simulink library "nmc"  (R2015b)
settings: Solver=ode45  SolverMode=SingleTasking  StartTime=0.0  StopTime=10.0  RelTol=1e-3
undefined symbols (not defined in the file): c, c_jointstop, CtrlPar_FP_List, CtrlPar_FP_R_List, CtrlPar_LL_List, CtrlPar_St_List, CtrlPar_St_R_List, CtrlPar_Sw_List, CtrlPar_Sw_R_List, CtrlPar_theta0_List, CtrlPar_Tr_List, CtrlPar_Tr_R_List, CtrlPar_VelocityFile_List, D1G_HAT, eref, FmaxBFSH, FmaxGAS, FmaxGLU, FmaxHAB, FmaxHAD, FmaxHAM, FmaxHFL, FmaxRF, FmaxSOL, FmaxTA, FmaxVAS, init_a_tgt, init_a_tgtR, K, leg_l, LongDelay, LongLoopDelay, loptBFSH, loptGAS, loptGLU, loptHAB, loptHAD, loptHAM, loptHFL, loptRF, loptSOL, loptTA, loptVAS, lslackBFSH, lslackGAS, lslackGLU, lslackHAB, lslackHAD, lslackHAM, lslackHFL, lslackRF, lslackSOL, lslackTA, lslackVAS, magnitude, maxLoad_control_List, MidDelay, N, phi12_LowLimit, phi12_UpLimit ... (+96)
libraries: nmc x63, simulink_extras x30, simulink x15, LopesDevelopmentLibrary x3
(part 1 of 10)
settings Model: Creator=efx  LastModifiedBy=brugtjh
settings DataIOCC: SaveFormat=Array
settings OptimizationCC: BlockReduction=off  BooleanDataType=off
settings DebuggingCC: SaveWithParameterizedLinksMsg=none  UnderspecifiedInitializationDetection=Classic  MergeDetectMultiDrivingBlocksExec=none  SignalResolutionControl=TryResolveAllWithWarning  StrictBusMsg=Warning
settings HardwareCC: ProdBitPerPointer=32  ProdLargestAtomicFloat=None  ProdIntDivRoundTo=Undefined  ProdEndianess=Unspecified  ProdWordSize=32  ProdHWDeviceType=32-bit Generic  TargetUnknown=on
settings GRTTargetCC: GeneratePreprocessorConditionals=Disable all
settings ConfigComp: CovModelRefEnable=Off  CovSFcnEnable=off

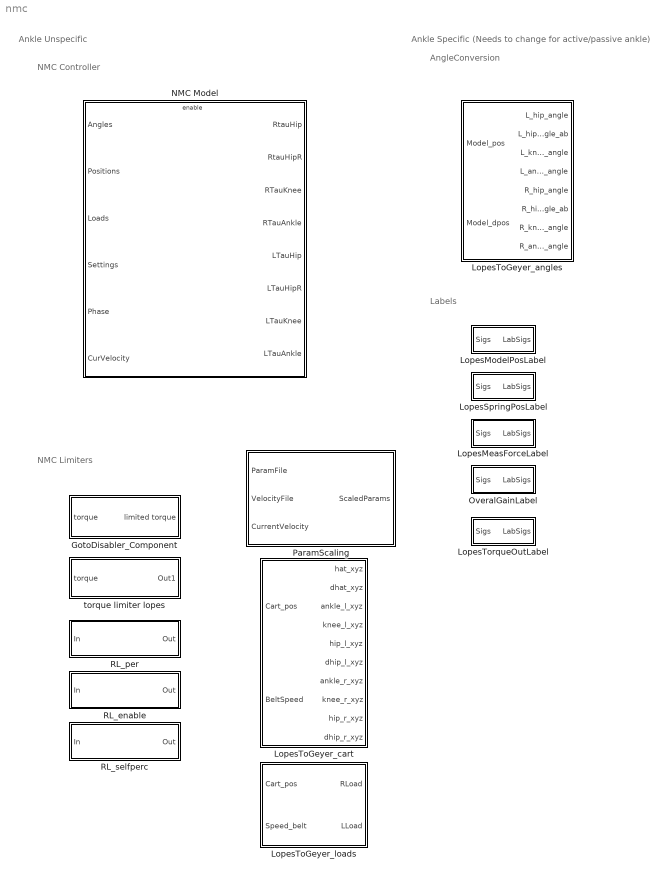
== system nmc ==
  note: Ankle Specific (Needs to change for active/passive ankle)
  note: AngleConversion
  note: NMC Limiters
  note: NMC Controller
  note: Ankle Unspecific
  note: Labels
  GotoDisabler_Component : Subsystem  mask{GotoTag=DisableNMC_Component}
      mask prompts: GotoTag "Simulink:blkprm_prompts:FromGotoTag"
      mask TypeOptions GotoTag: From/GotoTag
  LopesMeasForceLabel : Subsystem
  LopesModelPosLabel : Subsystem
  LopesSpringPosLabel : Subsystem
  LopesToGeyer_angles : Subsystem
  LopesToGeyer_cart : Subsystem
  LopesToGeyer_loads : Subsystem
  LopesTorqueOutLabel : Subsystem
  NMC Model : Subsystem
  OveralGainLabel : Subsystem
  ParamScaling : Subsystem
  RL_enable : Subsystem
  RL_per : Subsystem
  RL_selfperc : Subsystem
  torque limiter lopes : Subsystem  mask{TorqueLimiterPercentage=TorqueLimiterPercentage}
      mask prompts: TorqueLimiterPercentage "Simulink:blkprm_prompts:FromGotoTag"
      mask TypeOptions TorqueLimiterPercentage: From/GotoTag

== system nmc/GotoDisabler_Component ==
  torque : Inport
  Product : Product
  limited torque : Outport
  wires:
  torque/1 -> Product/2
  Product/1 -> limited torque/1
  [DisableNMC_Component] -> Product/1

== system nmc/LopesMeasForceLabel ==
  Sigs : Inport
  AnklePF : Concatenate  NumInputs=1
  Demux : Demux
  HipFlx : Concatenate  NumInputs=1
  KneeFlx : Concatenate  NumInputs=1
  MeasForce - HipAbd : Concatenate  NumInputs=1
  Mux : Mux
  LabSigs : Outport
  wires:
  Demux/3 -> KneeFlx/1
  Demux/2 -> HipFlx/1
  Demux/1 -> MeasForce - HipAbd/1
  HipFlx/1 -> Mux/2  "HipFlx"
  KneeFlx/1 -> Mux/3  "KneeFlx"
  MeasForce - HipAbd/1 -> Mux/1  "MeasForce - HipAbd"
  Sigs/1 -> Demux/1
  Mux/1 -> LabSigs/1
  Demux/4 -> AnklePF/1
  AnklePF/1 -> Mux/4  "AnklePF"

== system nmc/LopesModelPosLabel ==
  Sigs : Inport
  Angle - HipAbd : Concatenate  NumInputs=1
  AnklePF : Concatenate  NumInputs=1
  Demux : Demux
  HipFlx : Concatenate  NumInputs=1
  KneeFlx : Concatenate  NumInputs=1
  Mux : Mux
  LabSigs : Outport
  wires:
  Demux/3 -> KneeFlx/1
  Demux/2 -> HipFlx/1
  Demux/1 -> Angle - HipAbd/1
  HipFlx/1 -> Mux/2  "HipFlx"
  KneeFlx/1 -> Mux/3  "KneeFlx"
  Angle - HipAbd/1 -> Mux/1  "Angle - HipAbd"
  Sigs/1 -> Demux/1
  Mux/1 -> LabSigs/1
  Demux/4 -> AnklePF/1
  AnklePF/1 -> Mux/4  "AnklePF"

== system nmc/LopesSpringPosLabel ==
  Sigs : Inport
  AnklePF : Concatenate  NumInputs=1
  Demux : Demux
  HipFlx : Concatenate  NumInputs=1
  KneeFlx : Concatenate  NumInputs=1
  Mux : Mux
  SpringPos - HipAbd : Concatenate  NumInputs=1
  LabSigs : Outport
  wires:
  Demux/3 -> KneeFlx/1
  Demux/2 -> HipFlx/1
  Demux/1 -> SpringPos - HipAbd/1
  HipFlx/1 -> Mux/2  "HipFlx"
  KneeFlx/1 -> Mux/3  "KneeFlx"
  SpringPos - HipAbd/1 -> Mux/1  "SpringPos - HipAbd"
  Sigs/1 -> Demux/1
  Mux/1 -> LabSigs/1
  Demux/4 -> AnklePF/1
  AnklePF/1 -> Mux/4  "AnklePF"

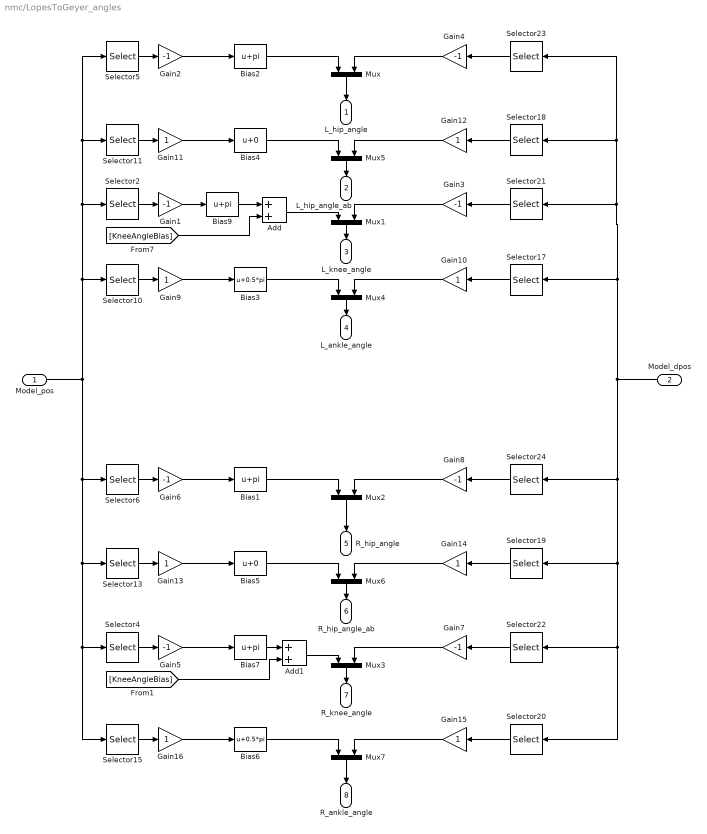
== system nmc/LopesToGeyer_angles ==
  Model_pos : Inport
  Model_dpos : Inport  Port=2
  Add : Sum
  Add1 : Sum
  Bias{1..2,7,9} (4 alike) : Bias  Bias=pi
  Bias3 : Bias  Bias=0.5*pi
  Bias4 : Bias
  Bias5 : Bias
  Bias6 : Bias  Bias=0.5*pi
  Gain{1..8} (8 alike) : Gain  Gain=-1
  Gain{9..16} (8 alike) : Gain
  Mux{,1..7} (8 alike) : Mux  Inputs=2
  Selector10 : Selector  InputPortWidth=SelectorLOPESModelPosSize  IndexOptions=Index vector (dialog)  Indices=[6]  OutputSizes=1
  Selector11 : Selector  InputPortWidth=SelectorLOPESModelPosSize  IndexOptions=Index vector (dialog)  Indices=[3]  OutputSizes=1
  Selector13 : Selector  InputPortWidth=SelectorLOPESModelPosSize  IndexOptions=Index vector (dialog)  Indices=[7]  OutputSizes=1
  Selector15 : Selector  InputPortWidth=SelectorLOPESModelPosSize  IndexOptions=Index vector (dialog)  Indices=[10]  OutputSizes=1
  Selector17 : Selector  InputPortWidth=SelectorLOPESModelPosSize  IndexOptions=Index vector (dialog)  Indices=[6]  OutputSizes=1
  Selector18 : Selector  InputPortWidth=SelectorLOPESModelPosSize  IndexOptions=Index vector (dialog)  Indices=[3]  OutputSizes=1
  Selector19 : Selector  InputPortWidth=SelectorLOPESModelPosSize  IndexOptions=Index vector (dialog)  Indices=[7]  OutputSizes=1
  Selector2 : Selector  InputPortWidth=SelectorLOPESModelPosSize  IndexOptions=Index vector (dialog)  Indices=[5]  OutputSizes=1
  Selector20 : Selector  InputPortWidth=SelectorLOPESModelPosSize  IndexOptions=Index vector (dialog)  Indices=[10]  OutputSizes=1
  Selector21 : Selector  InputPortWidth=SelectorLOPESModelPosSize  IndexOptions=Index vector (dialog)  Indices=[5]  OutputSizes=1
  Selector22 : Selector  InputPortWidth=SelectorLOPESModelPosSize  IndexOptions=Index vector (dialog)  Indices=[9]  OutputSizes=1
  Selector23 : Selector  InputPortWidth=SelectorLOPESModelPosSize  IndexOptions=Index vector (dialog)  Indices=[4]  OutputSizes=1
  Selector24 : Selector  InputPortWidth=SelectorLOPESModelPosSize  IndexOptions=Index vector (dialog)  Indices=[8]  OutputSizes=1
  Selector4 : Selector  InputPortWidth=SelectorLOPESModelPosSize  IndexOptions=Index vector (dialog)  Indices=[9]  OutputSizes=1
  Selector5 : Selector  InputPortWidth=SelectorLOPESModelPosSize  IndexOptions=Index vector (dialog)  Indices=[4]  OutputSizes=1
  Selector6 : Selector  InputPortWidth=SelectorLOPESModelPosSize  IndexOptions=Index vector (dialog)  Indices=[8]  OutputSizes=1
  L_hip_angle : Outport
  L_hip_angle_ab : Outport  Port=2
  L_knee_angle : Outport  Port=3
  L_ankle_angle : Outport  Port=4
  R_hip_angle : Outport  Port=5
  R_hip_angle_ab : Outport  Port=6
  R_knee_angle : Outport  Port=7
  R_ankle_angle : Outport  Port=8
  wires:
  Gain6/1 -> Bias1/1
  Selector6/1 -> Gain6/1
  Gain5/1 -> Bias7/1
  Selector4/1 -> Gain5/1
  Gain2/1 -> Bias2/1
  Selector5/1 -> Gain2/1
  Gain1/1 -> Bias9/1
  Selector2/1 -> Gain1/1
  Bias2/1 -> Mux/1
  Bias1/1 -> Mux2/1
  Selector24/1 -> Gain8/1
  Selector23/1 -> Gain4/1
  Selector21/1 -> Gain3/1
  Gain7/1 -> Mux3/2
  Gain4/1 -> Mux/2
  Gain3/1 -> Mux1/2
  Gain8/1 -> Mux2/2
  Selector22/1 -> Gain7/1
  Mux/1 -> L_hip_angle/1
  Mux1/1 -> L_knee_angle/1
  Mux2/1 -> R_hip_angle/1
  Mux3/1 -> R_knee_angle/1
  Gain9/1 -> Bias3/1
  Selector10/1 -> Gain9/1
  Selector17/1 -> Gain10/1
  Gain10/1 -> Mux4/2
  Gain11/1 -> Bias4/1
  Selector11/1 -> Gain11/1
  Bias4/1 -> Mux5/1
  Selector18/1 -> Gain12/1
  Gain12/1 -> Mux5/2
  Mux5/1 -> L_hip_angle_ab/1
  Gain13/1 -> Bias5/1
  Selector13/1 -> Gain13/1
  Bias5/1 -> Mux6/1
  Selector19/1 -> Gain14/1
  Gain14/1 -> Mux6/2
  Mux6/1 -> R_hip_angle_ab/1
  Model_pos/1 -> Selector2/1, Selector11/1, Selector5/1, Selector10/1, Selector6/1, Selector13/1, Selector15/1, Selector4/1
  Model_dpos/1 -> Selector24/1, Selector19/1, Selector20/1, Selector22/1, Selector17/1, Selector21/1, Selector23/1, Selector18/1
  Gain16/1 -> Bias6/1
  Selector15/1 -> Gain16/1
  Selector20/1 -> Gain15/1
  Gain15/1 -> Mux7/2
  Bias9/1 -> Add/1
  [KneeAngleBias] -> Add/2
  Add/1 -> Mux1/1
  [KneeAngleBias] -> Add1/2
  Bias7/1 -> Add1/1
  Add1/1 -> Mux3/1
  Mux4/1 -> L_ankle_angle/1
  Mux7/1 -> R_ankle_angle/1
  Bias6/1 -> Mux7/1
  Bias3/1 -> Mux4/1

== system nmc/LopesToGeyer_cart ==
  Cart_pos : Inport
  BeltSpeed : Inport  Port=2
  BeltSpeed1 : InportShadow  Port=2
  BeltSpeed2 : InportShadow  Port=2
  Constant : Constant  Value=theta0_control_List
  Constant1 : Constant  Value=CtrlPar_VelocityFile_List
  FilteredDerivative1 : LopesDevelopmentLibrary/Various/FilteredDerivative  w=7*(2*pi)  z=0.7
  FilteredDerivative2 : LopesDevelopmentLibrary/Various/FilteredDerivative  w=7*(2*pi)  z=0.7
  FilteredDerivative3 : LopesDevelopmentLibrary/Various/FilteredDerivative  w=7*(2*pi)  z=0.7
  ParamScaling : nmc/ParamScaling
  Selector1 : Selector  InputPortWidth=21  IndexOptions=Index vector (dialog)  Indices=[1 2 3]  OutputSizes=1
  Selector10 : Selector  InputPortWidth=21  IndexOptions=Index vector (dialog)  Indices=[16 17 18]  OutputSizes=1
  Selector11 : Selector  InputPortWidth=21  IndexOptions=Index vector (dialog)  Indices=[13 14 15]  OutputSizes=1
  Selector2 : Selector  InputPortWidth=7  IndexOptions=Index vector (dialog)  Indices=[2]  OutputSizes=1
  Selector3 : Selector  InputPortWidth=7  IndexOptions=Index vector (dialog)  Indices=[2]  OutputSizes=1
  Selector4 : Selector  InputPortWidth=7  IndexOptions=Index vector (dialog)  Indices=[2]  OutputSizes=1
  Selector5 : Selector  InputPortWidth=21  IndexOptions=Index vector (dialog)  Indices=[10 11 12]  OutputSizes=1
  Selector6 : Selector  InputPortWidth=21  IndexOptions=Index vector (dialog)  Indices=[7 8 9]  OutputSizes=1
  Selector7 : Selector  InputPortWidth=21  IndexOptions=Index vector (dialog)  Indices=[4 5 6]  OutputSizes=1
  Selector9 : Selector  InputPortWidth=21  IndexOptions=Index vector (dialog)  Indices=[19 20 21]  OutputSizes=1
  Subsystem : Subsystem
  Subsystem1 : Subsystem
  Subsystem2 : Subsystem
  Subsystem7 : Subsystem
  hat_xyz : Outport
  dhat_xyz : Outport  Port=2
  ankle_l_xyz : Outport  Port=3
  knee_l_xyz : Outport  Port=4
  hip_l_xyz : Outport  Port=5
  dhip_l_xyz : Outport  Port=6
  ankle_r_xyz : Outport  Port=7
  knee_r_xyz : Outport  Port=8
  hip_r_xyz : Outport  Port=9
  dhip_r_xyz : Outport  Port=10
  wires:
  Cart_pos/1 -> Selector10/1, Selector11/1, Selector9/1, Selector1/1, Selector5/1, Selector6/1, Selector7/1
  FilteredDerivative2/1 -> Subsystem7/1(1)
  FilteredDerivative1/1 -> Subsystem1/1(1)
  Selector6/1 -> knee_l_xyz/1
  Selector7/1 -> hip_l_xyz/1, FilteredDerivative1/1
  Selector5/1 -> ankle_l_xyz/1
  Selector9/1 -> ankle_r_xyz/1
  Selector10/1 -> knee_r_xyz/1
  Selector1/1 -> Subsystem/1(Pelvis_XYZ)
  Selector11/1 -> hip_r_xyz/1, FilteredDerivative3/1
  Subsystem7/1(2) -> dhat_xyz/1
  Subsystem1/1(2) -> dhip_l_xyz/1
  Subsystem2/1(2) -> dhip_r_xyz/1
  BeltSpeed/1 -> Selector4/1
  BeltSpeed1/1 -> Selector2/1
  Selector2/1 -> Subsystem1/2(BeltSpeed)
  BeltSpeed2/1 -> Selector3/1
  Selector3/1 -> Subsystem2/2(BeltSpeed)
  FilteredDerivative3/1 -> Subsystem2/1(1)
  Subsystem/1(HAT_XYZ) -> hat_xyz/1, FilteredDerivative2/1
  Constant/1 -> ParamScaling/1
  Constant1/1 -> ParamScaling/2
  Selector4/1 -> Subsystem7/2(BeltSpeed), ParamScaling/3
  ParamScaling/1 -> Subsystem/2(BodyAngle)

== system nmc/LopesToGeyer_loads ==
  Cart_pos : Inport
  "Speed_belt " : Inport  Port=2
  Add : Sum  Inputs=+-
  Add1 : Sum  Inputs=+-
  Add2 : Sum  Inputs=-+
  Bias : Bias  Bias=0.5*pi
  COPz : Selector  InputPortWidth=7  IndexOptions=Index vector (dialog)  Indices=[6]  OutputSizes=1
  Constant : Constant  Value=maxLoad_control_List
  Constant1 : Constant  Value=CtrlPar_VelocityFile_List
  Divide : Product  Inputs=**
  Divide1 : Product  Inputs=**
  Left_Ankle_z : Selector  InputPortWidth=21  IndexOptions=Index vector (dialog)  Indices=[12]  OutputSizes=1
  MeasuredSpeed : Selector  InputPortWidth=7  IndexOptions=Index vector (dialog)  Indices=[2]  OutputSizes=1
  ParamScaling : nmc/ParamScaling
  Right_Ankle_z : Selector  InputPortWidth=21  IndexOptions=Index vector (dialog)  Indices=[21]  OutputSizes=1
  SafeDivide : Subsystem
      mask Display:
      | port_label('input',1,'/')
      | port_label('input',2,'X')
      | port_label('output',1,'')
  SafeDivide1 : Subsystem
      mask Display:
      | port_label('input',1,'/')
      | port_label('input',2,'X')
      | port_label('output',1,'')
  Saturation : Saturate  UpperLimit=inf  LowerLimit=0
  Saturation1 : Saturate  UpperLimit=inf  LowerLimit=0
  "RLoad " : Outport
  LLoad : Outport  Port=2
  wires:
  Cart_pos/1 -> Left_Ankle_z/1, Right_Ankle_z/1
  "Speed_belt "/1 -> COPz/1, MeasuredSpeed/1
  Left_Ankle_z/1 -> Add1/1, Add/1
  Right_Ankle_z/1 -> Add2/1, Add/2
  COPz/1 -> Add2/2, Add1/2
  Add/1 -> SafeDivide1/1(Denominator), SafeDivide/1(Denominator)
  Add1/1 -> SafeDivide1/2(Numerator)
  SafeDivide1/1(Out) -> Divide/2
  SafeDivide/1(Out) -> Divide1/2
  Divide1/1 -> Saturation1/1
  Divide/1 -> Saturation/1
  Saturation/1 -> "RLoad "/1
  Saturation1/1 -> LLoad/1
  Add2/1 -> SafeDivide/2(Numerator)
  Constant/1 -> ParamScaling/1
  ParamScaling/1 -> Divide1/1, Divide/1
  Constant1/1 -> ParamScaling/2
  MeasuredSpeed/1 -> ParamScaling/3

== system nmc/LopesTorqueOutLabel ==
  Sigs : Inport
  AnklePF : Concatenate  NumInputs=1
  Demux : Demux
  HipFlx : Concatenate  NumInputs=1
  KneeFlx : Concatenate  NumInputs=1
  Mux : Mux
  TorqueOut - HipAbd : Concatenate  NumInputs=1
  LabSigs : Outport
  wires:
  Demux/3 -> KneeFlx/1
  Demux/2 -> HipFlx/1
  Demux/1 -> TorqueOut - HipAbd/1
  HipFlx/1 -> Mux/2  "HipFlx"
  KneeFlx/1 -> Mux/3  "KneeFlx"
  TorqueOut - HipAbd/1 -> Mux/1  "TorqueOut - HipAbd"
  Sigs/1 -> Demux/1
  Mux/1 -> LabSigs/1
  Demux/4 -> AnklePF/1
  AnklePF/1 -> Mux/4  "AnklePF"

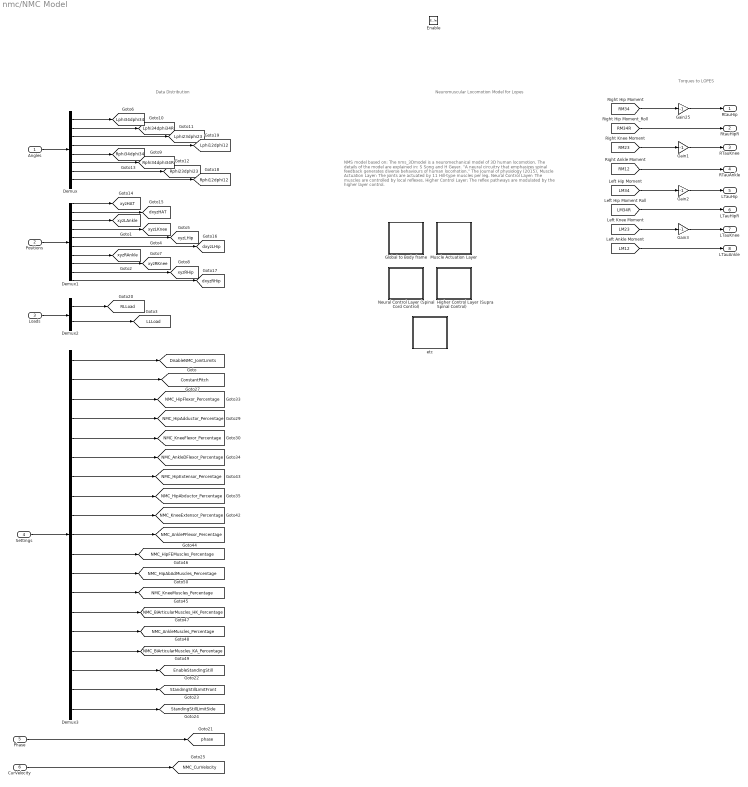
== system nmc/NMC Model ==
  note: Neuromuscular Locomotion Model for Lopes
  note: NMS model based on:
      | The nms_3Dmodel is a neuromechanical model of 3D human locomotion.
      | The details of the model are explained in:
      | S Song and H Geyer. "A neural circuitry that emphasizes spinal feedback
      | generates diverse behaviours of human locomotion." The Journal of physiology (2015).
      |
      | Muscle Actuation Layer:
      | The joints are actuated by 11 Hill-type muscles per leg.
      |
      | Neural Control Layer:
      | The muscles are controlled by local reflexes.
      |
      | Higher Control Layer:
      | The reflex pathways are modulated by the higher layer control.
  note: Data Distribution
  note: Torques to LOPES
  Angles : Inport
  Positions : Inport  Port=2
  Loads : Inport  Port=3
  Settings : Inport  Port=4
  Phase : Inport  Port=5
  CurVelocity : Inport  Port=6
  Enable : EnablePort  StatesWhenEnabling=reset
  Demux : Demux  Outputs=8
  Demux1 : Demux  Outputs=10
  Demux2 : Demux  Outputs=2
  Demux3 : Demux  Outputs=19
  Gain{1..3,25} (4 alike) : Gain  Gain=-1
  Global to Body frame : Subsystem
  Higher Control Layer (Supra Spinal Control) : Subsystem
  Muscle Actuation Layer : Subsystem
  Neural Control Layer (Spinal Cord Control) : Subsystem
  etc : Subsystem
  RtauHip : Outport
  RtauHipR : Outport  Port=2
  RTauKnee : Outport  Port=3
  RTauAnkle : Outport  Port=4
  LTauHip : Outport  Port=5
  LTauHipR : Outport  Port=6
  LTauKnee : Outport  Port=7
  LTauAnkle : Outport  Port=8
  tag scope: ConstantPitch=global, DisableNMC_JointLimits=global, EnableStandingStill=global, LLLoad=global, Lphi12dphi12=global, Lphi23dphi23=global, Lphi34dphi34=global, Lphi34dphi34R=global, NMC_AnkleDFlexor_Percentage=global, NMC_AnkleMuscles_Percentage=global, NMC_AnklePFlexor_Percentage=global, NMC_BiArticularMuscles_HK_Percentage=global, NMC_BiArticularMuscles_KA_Percentage=global, NMC_CurVelocity=global, NMC_HipAbAdMuscles_Percentage=global, NMC_HipAbductor_Percentage=global, NMC_HipAdductor_Percentage=global, NMC_HipExtensor_Percentage=global, NMC_HipFEMuscles_Percentage=global, NMC_HipFlexor_Percentage=global, NMC_KneeExtensor_Percentage=global, NMC_KneeFlexor_Percentage=global, NMC_KneeMuscles_Percentage=global, RLLoad=global, Rphi12dphi12=global, Rphi23dphi23=global, Rphi34dphi34=global, Rphi34dphi34R=global, StandingStillLimitFront=global, StandingStillLimitSide=global, dxyzHAT=global, dxyzLHip=global, dxyzRHip=global, phase=global, xyzHAT=global, xyzLAnkle=global, xyzLHip=global, xyzLKnee=global, xyzRAnkle=global, xyzRHip=global, xyzRKnee=global
  wires:
  [RM34] -> Gain25/1
  [RM23] -> Gain1/1
  [LM34] -> Gain2/1
  [LM23] -> Gain3/1
  Angles/1 -> Demux/1
  Demux/1 -> [Lphi34dphi34]
  Demux/5 -> [Rphi34dphi34]
  Demux/6 -> [Rphi34dphi34R]
  Demux/7 -> [Rphi23dphi23]
  Demux/8 -> [Rphi12dphi12]
  Demux/2 -> [Lphi34dphi34R]
  Demux/3 -> [Lphi23dphi23]
  Demux/4 -> [Lphi12dphi12]
  Positions/1 -> Demux1/1
  Demux1/1 -> [xyzHAT]
  Demux1/2 -> [dxyzHAT]
  Loads/1 -> Demux2/1
  Demux2/1 -> [RLLoad]
  Demux2/2 -> [LLLoad]
  Demux1/3 -> [xyzLAnkle]
  Demux1/4 -> [xyzLKnee]
  Demux1/5 -> [xyzLHip]
  Demux1/6 -> [dxyzLHip]
  Demux1/7 -> [xyzRAnkle]
  Demux1/8 -> [xyzRKnee]
  Demux1/9 -> [xyzRHip]
  Demux1/10 -> [dxyzRHip]
  [RM34R] -> RtauHipR/1
  [RM12] -> RTauAnkle/1
  [LM34R] -> LTauHipR/1
  [LM12] -> LTauAnkle/1
  Phase/1 -> [phase]
  Settings/1 -> Demux3/1
  Demux3/2 -> [ConstantPitch]
  Demux3/1 -> [DisableNMC_JointLimits]
  Demux3/15 -> [NMC_AnkleMuscles_Percentage]
  Demux3/13 -> [NMC_KneeMuscles_Percentage]
  Demux3/14 -> [NMC_BiArticularMuscles_HK_Percentage]
  Demux3/16 -> [NMC_BiArticularMuscles_KA_Percentage]
  Demux3/12 -> [NMC_HipAbAdMuscles_Percentage]
  Demux3/11 -> [NMC_HipFEMuscles_Percentage]
  Demux3/10 -> [NMC_AnklePFlexor_Percentage]
  Demux3/9 -> [NMC_KneeExtensor_Percentage]
  Demux3/8 -> [NMC_HipAbductor_Percentage]
  Demux3/7 -> [NMC_HipExtensor_Percentage]
  Demux3/6 -> [NMC_AnkleDFlexor_Percentage]
  Demux3/5 -> [NMC_KneeFlexor_Percentage]
  Demux3/4 -> [NMC_HipAdductor_Percentage]
  Demux3/3 -> [NMC_HipFlexor_Percentage]
  Gain25/1 -> RtauHip/1
  Gain1/1 -> RTauKnee/1
  Gain2/1 -> LTauHip/1
  Gain3/1 -> LTauKnee/1
  Demux3/17 -> [EnableStandingStill]
  Demux3/18 -> [StandingStillLimitFront]
  Demux3/19 -> [StandingStillLimitSide]
  CurVelocity/1 -> [NMC_CurVelocity]

== system nmc/OveralGainLabel ==
  Sigs : Inport
  AnklePF : Concatenate  NumInputs=1
  Demux : Demux
  HipFlx : Concatenate  NumInputs=1
  KneeFlx : Concatenate  NumInputs=1
  Mux : Mux
  OveralGain - HipAbd : Concatenate  NumInputs=1
  LabSigs : Outport
  wires:
  Demux/3 -> KneeFlx/1
  Demux/2 -> HipFlx/1
  Demux/1 -> OveralGain - HipAbd/1
  HipFlx/1 -> Mux/2  "HipFlx"
  KneeFlx/1 -> Mux/3  "KneeFlx"
  OveralGain - HipAbd/1 -> Mux/1  "OveralGain - HipAbd"
  Sigs/1 -> Demux/1
  Mux/1 -> LabSigs/1
  Demux/4 -> AnklePF/1
  AnklePF/1 -> Mux/4  "AnklePF"

== system nmc/ParamScaling ==
  ParamFile : Inport
  VelocityFile : Inport  Port=2
  CurrentVelocity : Inport  Port=3
  ScalerFull : MATLAB Function
      settings: MinAlgLoopOccurrences=on
  ScaledParams : Outport
  wires:
  ScalerFull/1(ScaledParam) -> ScaledParams/1
  ParamFile/1 -> ScalerFull/1(ParamFile)
  VelocityFile/1 -> ScalerFull/2(VelocityFile)
  CurrentVelocity/1 -> ScalerFull/3(Velocity)

== system nmc/RL_enable ==
  In : Inport
  Gain : Gain  Gain=-1
  Gain1 : Gain  Gain=0.01
  Rate Limiter Dynamic : simulink/Discontinuities/Rate Limiter Dynamic
  Out : Outport
  wires:
  Gain1/1 -> Rate Limiter Dynamic/1, Gain/1
  Gain/1 -> Rate Limiter Dynamic/3
  [RateLimiterPercentage] -> Gain1/1
  In/1 -> Rate Limiter Dynamic/2
  Rate Limiter Dynamic/1 -> Out/1

== system nmc/RL_per ==
  In : Inport
  Gain : Gain  Gain=-1
  Rate Limiter Dynamic : simulink/Discontinuities/Rate Limiter Dynamic
  Out : Outport
  wires:
  Rate Limiter Dynamic/1 -> Out/1
  In/1 -> Rate Limiter Dynamic/2
  [RateLimiterPercentage] -> Gain/1, Rate Limiter Dynamic/1
  Gain/1 -> Rate Limiter Dynamic/3

== system nmc/RL_selfperc ==
  In : Inport
  Constant : Constant  Value=0
  Gain : Gain  Gain=-1
  MinMax Running Resettable : simulink/Math Operations/MinMax Running Resettable  Function=max  vinit=0.0
  PercToPoint : Gain  Gain=0.01
  Product : Product
  Rate Limiter Dynamic : simulink/Discontinuities/Rate Limiter Dynamic
  Out : Outport
  wires:
  Constant/1 -> MinMax Running Resettable/2
  MinMax Running Resettable/1 -> Rate Limiter Dynamic/1, Gain/1
  Gain/1 -> Rate Limiter Dynamic/3
  In/1 -> Product/2, Rate Limiter Dynamic/2
  Rate Limiter Dynamic/1 -> Out/1
  [RateLimiterPercentage] -> PercToPoint/1
  PercToPoint/1 -> Product/1
  Product/1 -> MinMax Running Resettable/1

== system nmc/torque limiter lopes ==
  torque : Inport
  Gain1 : Gain  Gain=0.01
  Product1 : Product
  Out1 : Outport
  wires:
  Product1/1 -> Out1/1
  torque/1 -> Product1/2
  [TorqueLimiterPercentage] -> Gain1/1
  Gain1/1 -> Product1/1

== system nmc/LopesToGeyer_cart/Subsystem ==
  Pelvis_XYZ : Inport
  BodyAngle : Inport  Port=2
  Add : Sum
  Add1 : Sum
  Demux : Demux  Outputs=3
  Gain : Gain  Gain=D1G_HAT
  Gain1 : Gain
  Gain2 : Gain  Gain=D1G_HAT
  Mux : Mux  Inputs=3
  Trigonometric Function : Trigonometry
  Trigonometric Function1 : Trigonometry  Operator=cos
  HAT_XYZ : Outport
  wires:
  Mux/1 -> HAT_XYZ/1
  Add1/1 -> Mux/2
  Demux/3 -> Gain1/1
  Pelvis_XYZ/1 -> Demux/1
  Demux/2 -> Add1/2
  Demux/1 -> Add/2
  Gain1/1 -> Mux/3
  Add/1 -> Mux/1
  BodyAngle/1 -> Trigonometric Function1/1, Trigonometric Function/1
  Trigonometric Function/1 -> Gain/1
  Gain/1 -> Add/1
  Trigonometric Function1/1 -> Gain2/1
  Gain2/1 -> Add1/1

== system nmc/LopesToGeyer_cart/Subsystem1 ==
  1 : Inport
  BeltSpeed : Inport  Port=2
  Add : Sum
  Demux : Demux  Outputs=3
  Mux : Mux  Inputs=3
  2 : Outport
  wires:
  Demux/3 -> Mux/3
  Demux/1 -> Add/2
  1/1 -> Demux/1
  Demux/2 -> Mux/2
  Mux/1 -> 2/1
  BeltSpeed/1 -> Add/1
  Add/1 -> Mux/1

== system nmc/LopesToGeyer_cart/Subsystem2 ==
  1 : Inport
  BeltSpeed : Inport  Port=2
  Add : Sum
  Demux : Demux  Outputs=3
  Mux : Mux  Inputs=3
  2 : Outport
  wires:
  Demux/3 -> Mux/3
  Demux/1 -> Add/2
  1/1 -> Demux/1
  Demux/2 -> Mux/2
  Mux/1 -> 2/1
  BeltSpeed/1 -> Add/1
  Add/1 -> Mux/1

== system nmc/LopesToGeyer_cart/Subsystem7 ==
  1 : Inport
  BeltSpeed : Inport  Port=2
  Add : Sum
  Demux : Demux  Outputs=3
  Mux : Mux  Inputs=3
  2 : Outport
  wires:
  Demux/3 -> Mux/3
  Demux/1 -> Add/2
  1/1 -> Demux/1
  Demux/2 -> Mux/2
  Mux/1 -> 2/1
  BeltSpeed/1 -> Add/1
  Add/1 -> Mux/1

== system nmc/LopesToGeyer_loads/SafeDivide ==
  note: This block guarantees division-by-zero-free division.
  Denominator : Inport
  Numerator : Inport  Port=2
  Add : Sum
  Divide : Product  Inputs=*/
  Gain : Gain  Gain=1e-100
  Sign : Signum
  Out : Outport
  wires:
  Divide/1 -> Out/1
  Numerator/1 -> Divide/1
  Denominator/1 -> Add/1, Sign/1
  Add/1 -> Divide/2
  Sign/1 -> Gain/1
  Gain/1 -> Add/2

== system nmc/LopesToGeyer_loads/SafeDivide1 ==
  note: This block guarantees division-by-zero-free division.
  Denominator : Inport
  Numerator : Inport  Port=2
  Add : Sum
  Divide : Product  Inputs=*/
  Gain : Gain  Gain=1e-100
  Sign : Signum
  Out : Outport
  wires:
  Gain/1 -> Add/2
  Sign/1 -> Gain/1
  Add/1 -> Divide/2
  Denominator/1 -> Sign/1, Add/1
  Numerator/1 -> Divide/1
  Divide/1 -> Out/1

== system nmc/NMC Model/Global to Body frame ==
  note: Global to Body Frame Mapping
  Constant : Constant  Value=theta0_control_List
  Constant{1..4} (4 alike) : Constant  Value=0
  Constant20 : Constant  Value=CtrlPar_VelocityFile_List
  L GLU Golgi Tendon Organs5 : Gain  Gain=-1
  ParamScaling : nmc/ParamScaling
  Selector{3..4,8..9,11..14} (8 alike) : Selector  InputPortWidth=3  IndexOptions=Index vector (dialog)  Indices=[1 3]  OutputSizes=1
  Switch{,1..4} (5 alike) : Switch  Criteria=u2 ~= 0
  body pitch/roll/yaw in body frame --- x-axis: forward y-axis: leftward z-axis: parallel to gravity : Subsystem
  "lateral d, v in body frame (left)" : Subsystem
  "lateral d, v in body frame (right)" : Subsystem
  "sagittal d, v in body frame (left)" : Subsystem
  "sagittal d, v in body frame (right)" : Subsystem
  tag scope: dtheta=global, dthetaR=global, front_dv_L=global, front_dv_R=global, side_dv_L=global, side_dv_R=global, theta=global, thetaR=global, thetaY=global
  wires:
  Constant1/1 -> Switch1/1
  [xyzLAnkle] -> Selector9/1
  [xyzRAnkle] -> Selector11/1
  [dxyzHAT] -> Selector4/1
  Selector11/1 -> "lateral d, v in body frame (left)"/2(d0)
  Selector3/1 -> "lateral d, v in body frame (left)"/3(dist), "lateral d, v in body frame (right)"/3(dist)
  Selector4/1 -> "lateral d, v in body frame (left)"/4(vel), "lateral d, v in body frame (right)"/4(vel)
  [thetaY] -> "lateral d, v in body frame (left)"/1(body yaw), "lateral d, v in body frame (right)"/1(body yaw)
  [xyzHAT] -> Selector3/1
  Selector9/1 -> "lateral d, v in body frame (right)"/2(d0)
  [xyzLHip] -> body pitch/roll/yaw in body frame --- x-axis: forward y-axis: leftward z-axis: parallel to gravity/1(LHip)
  [dxyzLHip] -> body pitch/roll/yaw in body frame --- x-axis: forward y-axis: leftward z-axis: parallel to gravity/2(dLHip)
  [xyzRHip] -> body pitch/roll/yaw in body frame --- x-axis: forward y-axis: leftward z-axis: parallel to gravity/5(RHip)
  [dxyzRHip] -> body pitch/roll/yaw in body frame --- x-axis: forward y-axis: leftward z-axis: parallel to gravity/6(dRHip)
  [xyzHAT] -> body pitch/roll/yaw in body frame --- x-axis: forward y-axis: leftward z-axis: parallel to gravity/3(HAT)
  [dxyzHAT] -> body pitch/roll/yaw in body frame --- x-axis: forward y-axis: leftward z-axis: parallel to gravity/4(dHAT)
  "lateral d, v in body frame (left)"/1("d, v") -> L GLU Golgi Tendon Organs5/1
  [xyzLAnkle] -> Selector13/1
  [xyzRAnkle] -> Selector14/1
  [dxyzHAT] -> Selector12/1
  Selector14/1 -> "sagittal d, v in body frame (left)"/2(d0)
  Selector8/1 -> "sagittal d, v in body frame (left)"/3(dist), "sagittal d, v in body frame (right)"/3(dist)
  Selector12/1 -> "sagittal d, v in body frame (left)"/4(vel), "sagittal d, v in body frame (right)"/4(vel)
  [thetaY] -> "sagittal d, v in body frame (left)"/1(body yaw), "sagittal d, v in body frame (right)"/1(body yaw)
  [xyzHAT] -> Selector8/1
  Selector13/1 -> "sagittal d, v in body frame (right)"/2(d0)
  "sagittal d, v in body frame (left)"/1("d, v") -> [front_dv_L]
  "sagittal d, v in body frame (right)"/1("d, v") -> [front_dv_R]
  L GLU Golgi Tendon Organs5/1 -> [side_dv_L]
  "lateral d, v in body frame (right)"/1("d, v") -> [side_dv_R]
  body pitch/roll/yaw in body frame --- x-axis: forward y-axis: leftward z-axis: parallel to gravity/1(th_pitch) -> Switch/3
  body pitch/roll/yaw in body frame --- x-axis: forward y-axis: leftward z-axis: parallel to gravity/2(dth_pitch) -> Switch1/3
  Switch/1 -> [theta]
  Switch1/1 -> [dtheta]
  [ConstantPitch] -> Switch4/2, Switch3/2, Switch2/2, Switch1/2, Switch/2
  body pitch/roll/yaw in body frame --- x-axis: forward y-axis: leftward z-axis: parallel to gravity/3(th_roll) -> Switch2/3
  Switch2/1 -> [thetaR]
  body pitch/roll/yaw in body frame --- x-axis: forward y-axis: leftward z-axis: parallel to gravity/4(dth_roll) -> Switch3/3
  Switch3/1 -> [dthetaR]
  body pitch/roll/yaw in body frame --- x-axis: forward y-axis: leftward z-axis: parallel to gravity/5(yaw) -> Switch4/3
  Switch4/1 -> [thetaY]
  Constant2/1 -> Switch2/1
  Constant3/1 -> Switch3/1
  Constant4/1 -> Switch4/1
  ParamScaling/1 -> Switch/1
  [NMC_CurVelocity] -> ParamScaling/3
  Constant20/1 -> ParamScaling/2
  Constant/1 -> ParamScaling/1

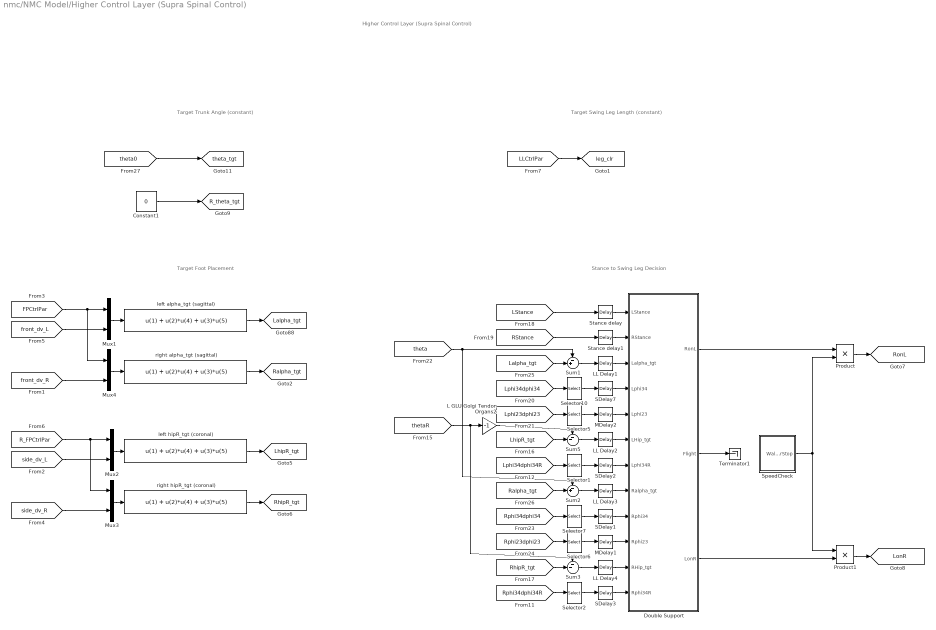
== system nmc/NMC Model/Higher Control Layer (Supra Spinal Control) ==
  note: Target Foot Placement
  note: Target Swing Leg Length
      | (constant)
  note: Stance to Swing Leg Decision
  note: Target Trunk Angle
      | (constant)
  note: Higher Control Layer
      | (Supra Spinal Control)
  Constant1 : Constant  Value=0
  Double Support : Subsystem
  L GLU Golgi Tendon Organs2 : Gain  Gain=-1
  LL Delay1 : TransportDelay  DelayTime=LongLoopDelay/2  InitialOutput=init_a_tgt
  LL Delay2 : TransportDelay  DelayTime=LongLoopDelay/2
  LL Delay3 : TransportDelay  DelayTime=LongLoopDelay/2  InitialOutput=init_a_tgt
  LL Delay4 : TransportDelay  DelayTime=LongLoopDelay/2
  MDelay1 : TransportDelay  DelayTime=MidDelay
  MDelay2 : TransportDelay  DelayTime=MidDelay
  Mux{1..4} (4 alike) : Mux  Inputs=2
  Product : Product
  Product1 : Product
  SDelay{1..3,7} (4 alike) : TransportDelay  DelayTime=ShortDelay
  Selector{1..2,5..7,10} (6 alike) : Selector  InputPortWidth=2  IndexOptions=Index vector (dialog)  Indices=1  OutputSizes=1
  SpeedCheck : Subsystem
  Stance delay : TransportDelay  DelayTime=MidDelay
  Stance delay1 : TransportDelay  DelayTime=MidDelay
  Sum1 : Sum  Inputs=-+|
  Sum2 : Sum  Inputs=-+|
  Sum3 : Sum  Inputs=--|
  Sum5 : Sum  Inputs=--|
  Terminator1 : Terminator
  left alpha_tgt (sagittal) : Fcn  Expr=u(1) + u(2)*u(4) + u(3)*u(5)
  left hipR_tgt (coronal) : Fcn  Expr=u(1) + u(2)*u(4) + u(3)*u(5)
  right alpha_tgt (sagittal) : Fcn  Expr=u(1) + u(2)*u(4) + u(3)*u(5)
  right hipR_tgt (coronal) : Fcn  Expr=u(1) + u(2)*u(4) + u(3)*u(5)
  tag scope: Lalpha_tgt=global, LhipR_tgt=global, LonR=global, R_theta_tgt=global, Ralpha_tgt=global, RhipR_tgt=global, RonL=global, leg_clr=global, theta_tgt=global
  wires:
  left alpha_tgt (sagittal)/1 -> [Lalpha_tgt]
  right alpha_tgt (sagittal)/1 -> [Ralpha_tgt]
  left hipR_tgt (coronal)/1 -> [LhipR_tgt]
  right hipR_tgt (coronal)/1 -> [RhipR_tgt]
  [LLCtrlPar] -> [leg_clr]
  [Lphi34dphi34] -> Selector10/1
  [Lphi23dphi23] -> Selector5/1
  Selector10/1 -> SDelay7/1
  Selector5/1 -> MDelay2/1
  [Rphi34dphi34] -> Selector7/1
  [Rphi23dphi23] -> Selector6/1
  Selector7/1 -> SDelay1/1
  Selector6/1 -> MDelay1/1
  Stance delay/1 -> Double Support/1(LStance)
  Stance delay1/1 -> Double Support/2(RStance)
  Double Support/1(RonL) -> Product/1
  [LStance] -> Stance delay/1
  [RStance] -> Stance delay1/1
  Double Support/2(Flight) -> Terminator1/1
  LL Delay1/1 -> Double Support/3(Lalpha_tgt)
  LL Delay3/1 -> Double Support/8(Ralpha_tgt)
  SDelay7/1 -> Double Support/4(Lphi34)
  SDelay1/1 -> Double Support/9(Rphi34)
  MDelay2/1 -> Double Support/5(Lphi23)
  MDelay1/1 -> Double Support/10(Rphi23)
  Sum1/1 -> LL Delay1/1
  [Lalpha_tgt] -> Sum1/2
  [theta] -> Sum1/1, Sum2/1
  [Ralpha_tgt] -> Sum2/2
  Sum2/1 -> LL Delay3/1
  [Lphi34dphi34R] -> Selector1/1
  Selector1/1 -> SDelay2/1
  SDelay2/1 -> Double Support/7(Lphi34R)
  LL Delay2/1 -> Double Support/6(LHip_tgt)
  Sum5/1 -> LL Delay2/1
  [LhipR_tgt] -> Sum5/2
  [thetaR] -> L GLU Golgi Tendon Organs2/1, Sum3/1
  L GLU Golgi Tendon Organs2/1 -> Sum5/1
  [Rphi34dphi34R] -> Selector2/1
  Selector2/1 -> SDelay3/1
  SDelay3/1 -> Double Support/12(Rphi34R)
  LL Delay4/1 -> Double Support/11(RHip_tgt)
  Sum3/1 -> LL Delay4/1
  [RhipR_tgt] -> Sum3/2
  [theta0] -> [theta_tgt]
  Constant1/1 -> [R_theta_tgt]
  Mux1/1 -> left alpha_tgt (sagittal)/1
  [FPCtrlPar] -> Mux4/1, Mux1/1
  [front_dv_L] -> Mux1/2
  Mux4/1 -> right alpha_tgt (sagittal)/1
  [front_dv_R] -> Mux4/2
  Mux2/1 -> left hipR_tgt (coronal)/1
  Mux3/1 -> right hipR_tgt (coronal)/1
  [R_FPCtrlPar] -> Mux3/1, Mux2/1
  [side_dv_L] -> Mux2/2
  [side_dv_R] -> Mux3/2
  Double Support/3(LonR) -> Product1/2
  Product1/1 -> [LonR]
  Product/1 -> [RonL]
  SpeedCheck/1(WalkOrStop) -> Product/2, Product1/1
